simulink model "sampleModel1473"  (R2023a)
settings: Solver=VariableStepAuto  StartTime=0.0  StopTime=10.0  RelTol=1e-3
libraries: hdlsllib x6, simulink x1
settings Model: Creator=user1  LastModifiedBy=user1

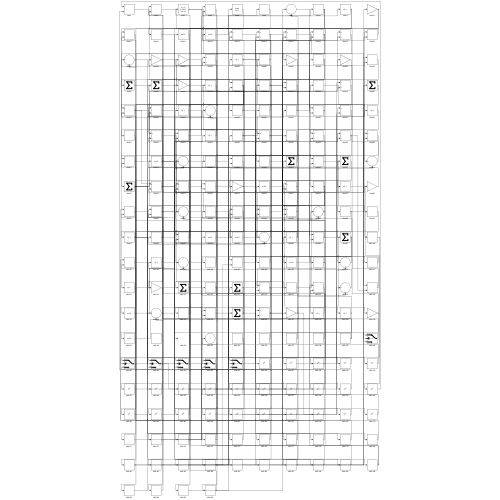
[thumbnail: Simulink's stored preview of the top-level diagram]
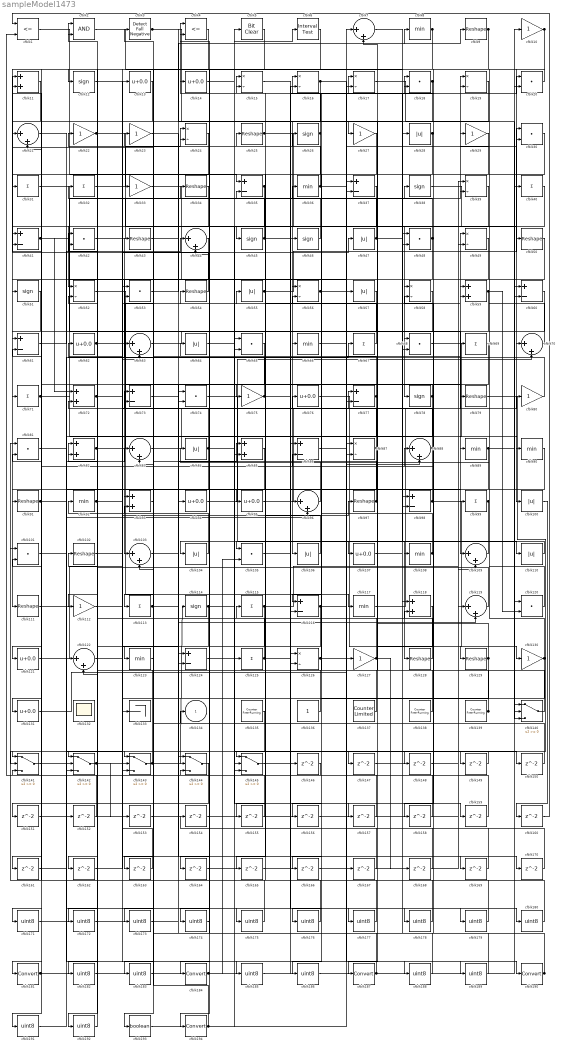
== system sampleModel1473 ==
  cfblk1 : RelationalOperator  Operator=<=  OutDataTypeStr=boolean  InputSameDT=off
  cfblk{10,22..23,27,29,33,75,80,112,127,130} (11 alike) : Gain
  cfblk{28,47,55,57,64,84,100,104,106,110} (10 alike) : Abs  SaturateOnIntegerOverflow=off
  cfblk{18,20,30,42,48,53,65,68,74,81,101,105,120} (13 alike) : DotProduct  OutDataTypeStr=Inherit: Inherit via internal rule
  cfblk{9,25,34,43,50,54,79,91,97,102,111,128..129} (13 alike) : Reshape
  cfblk{7,21,44,63,70,83,88,96,103,109,119,122} (12 alike) : Sum  Inputs=|++
  cfblk{13..14,62,76,94..95,107,121,131} (9 alike) : Bias  Bias=0.0  SaturateOnIntegerOverflow=off
  cfblk{8,36,66,89..90,92,108,117,123} (9 alike) : MinMax
  cfblk{11,59,72,82,85,93,118} (7 alike) : Sum
  cfblk{31..32,40,67,69,71,99,113,115,125} (10 alike) : Sum  Inputs=+
  cfblk{12,26,38,45..46,51,78,114} (8 alike) : Signum
  cfblk{35,37,41,60..61,73,77,86,98,116,124} (11 alike) : Sum  Inputs=+-
  cfblk{15..17,19,24,39,49,52,56,58,87,126} (12 alike) : Product  Inputs=*/  RndMeth=Zero  SaturateOnIntegerOverflow=on
  cfblk132 : Scope
      settings: Floating=on
  cfblk133 : Terminator
  cfblk135 : hdlsllib/Sources/Counter Free-Running  NumBits=16  tsamp=-1
  cfblk136 : Constant  SampleTime=-1
  cfblk137 : hdlsllib/Sources/Counter Limited  uplimit=7  tsamp=-1
  cfblk138 : hdlsllib/Sources/Counter Free-Running  NumBits=16  tsamp=-1
  cfblk139 : hdlsllib/Sources/Counter Free-Running  NumBits=16  tsamp=-1
  cfblk{140..145} (6 alike) : Switch  SaturateOnIntegerOverflow=off  InputSameDT=off
  cfblk{146..170} (25 alike) : Delay  SampleTime=1
  cfblk{171..180,182..183,185..186,188..189,191..192} (18 alike) : DataTypeConversion  OutDataTypeStr=uint8  SaturateOnIntegerOverflow=off  RndMeth=Floor
  cfblk{181,184,187,190,194} (5 alike) : DataTypeConversion  SaturateOnIntegerOverflow=off  RndMeth=Floor
  cfblk193 : DataTypeConversion  OutDataTypeStr=boolean  SaturateOnIntegerOverflow=off  RndMeth=Floor
  cfblk2 : Logic  AllPortsSameDT=off  OutDataTypeStr=boolean
  cfblk3 : hdlsllib/Logic and Bit Operations/Detect Fall Negative  vinit=0  OutDataTypeStr=boolean
  cfblk4 : RelationalOperator  Operator=<=  OutDataTypeStr=boolean  InputSameDT=off
  cfblk5 : simulink/Logic and Bit Operations/Bit Clear  iBit=0
      settings: LibrarySourceBlock=|
      | hdlsllib/Logic and Bit
      | Operations/Bit Clear
  cfblk6 : hdlsllib/Logic and Bit Operations/Interval Test  IntervalClosedRight=on  uplimit=0.5  IntervalClosedLeft=on  lowlimit=-0.5  OutDataTypeStr=boolean
  cfblk134 : Outport  VectorParamsAs1DForOutWhenUnconnected=off
  wires:
  cfblk76/1 -> cfblk129/1
  cfblk26/1 -> cfblk111/1, cfblk4/2
  cfblk110/1 -> cfblk104/1
  cfblk42/1 -> cfblk19/1
  cfblk32/1 -> cfblk24/1
  cfblk1/1 -> cfblk35/1
  cfblk8/1 -> cfblk71/1, cfblk174/1, cfblk193/1
  cfblk28/1 -> cfblk105/1, cfblk164/1
  cfblk80/1 -> cfblk43/1
  cfblk79/1 -> cfblk142/1
  cfblk72/1 -> cfblk13/1, cfblk177/1
  cfblk71/1 -> cfblk38/1, cfblk55/1, cfblk98/1, cfblk98/2
  cfblk19/1 -> cfblk106/1
  cfblk52/1 -> cfblk117/1
  cfblk139/1 -> cfblk77/1, cfblk16/1
  cfblk39/1 -> cfblk78/1
  cfblk54/1 -> cfblk11/1
  cfblk63/1 -> cfblk68/1
  cfblk44/1 -> cfblk103/1
  cfblk70/1 -> cfblk15/1
  cfblk96/1 -> cfblk22/1
  cfblk35/1 -> cfblk141/1, cfblk145/3, cfblk121/1
  cfblk29/1 -> cfblk45/1
  cfblk131/1 -> cfblk57/1
  cfblk2/1 -> cfblk48/1
  cfblk3/1 -> cfblk48/2, cfblk27/1
  cfblk14/1 -> cfblk8/1
  cfblk83/1 -> cfblk49/1
  cfblk106/1 -> cfblk15/2
  cfblk11/1 -> cfblk31/1
  cfblk85/1 -> cfblk91/1
  cfblk136/1 -> cfblk102/1
  cfblk98/1 -> cfblk130/1, cfblk11/2
  cfblk88/1 -> cfblk17/1, cfblk86/2
  cfblk77/1 -> cfblk21/1, cfblk116/2
  cfblk75/1 -> cfblk62/1, cfblk59/2, cfblk95/1
  cfblk145/1 -> cfblk46/1
  cfblk10/1 -> cfblk100/1, cfblk143/2
  cfblk97/1 -> cfblk93/1, cfblk36/1
  cfblk59/1 -> cfblk131/1, cfblk120/2
  cfblk65/1 -> cfblk181/1
  cfblk50/1 -> cfblk107/1
  cfblk87/1 -> cfblk24/2, cfblk192/1
  cfblk5/1 -> cfblk194/1
  cfblk118/1 -> cfblk187/1
  cfblk56/1 -> cfblk88/2, cfblk149/1
  cfblk58/1 -> cfblk113/1
  cfblk95/1 -> cfblk80/1
  cfblk82/1 -> cfblk54/1, cfblk76/1
  cfblk62/1 -> cfblk74/2, cfblk124/2, cfblk140/3
  cfblk78/1 -> cfblk142/2, cfblk75/1, cfblk87/2, cfblk155/1
  cfblk24/1 -> cfblk142/3
  cfblk22/1 -> cfblk127/1, cfblk112/1
  cfblk57/1 -> cfblk66/1
  cfblk143/1 -> cfblk114/1, cfblk42/2
  cfblk104/1 -> cfblk92/1
  cfblk60/1 -> cfblk184/1
  cfblk67/1 -> cfblk25/1
  cfblk41/1 -> cfblk109/1, cfblk72/1
  cfblk142/1 -> cfblk153/1, cfblk189/1
  cfblk129/1 -> cfblk7/2, cfblk156/1
  cfblk25/1 -> cfblk70/1, cfblk18/1
  cfblk114/1 -> cfblk6/1, cfblk162/1
  cfblk141/1 -> cfblk83/1
  cfblk47/1 -> cfblk19/2, cfblk34/1
  cfblk122/1 -> cfblk190/1
  cfblk33/1 -> cfblk87/1
  cfblk51/1 -> cfblk61/1
  cfblk117/1 -> cfblk10/1
  cfblk135/1 -> cfblk145/1
  cfblk130/1 -> cfblk29/1, cfblk140/2
  cfblk123/1 -> cfblk73/1
  cfblk68/1 -> cfblk90/1
  cfblk12/1 -> cfblk133/1
  cfblk102/1 -> cfblk59/1
  cfblk74/1 -> cfblk128/1
  cfblk128/1 -> cfblk63/1
  cfblk107/1 -> cfblk28/1
  cfblk17/1 -> cfblk120/1
  cfblk55/1 -> cfblk30/1, cfblk180/1
  cfblk94/1 -> cfblk70/2
  cfblk53/1 -> cfblk9/1
  cfblk34/1 -> cfblk52/1
  cfblk125/1 -> cfblk14/1, cfblk159/1
  cfblk13/1 -> cfblk51/1
  cfblk105/1 -> cfblk20/1
  cfblk73/1 -> cfblk79/1
  cfblk89/1 -> cfblk40/1, cfblk126/2
  cfblk49/1 -> cfblk58/1
  cfblk126/1 -> cfblk30/2, cfblk188/1
  cfblk138/1 -> cfblk64/1
  cfblk61/1 -> cfblk44/1
  cfblk140/1 -> cfblk26/1
  cfblk113/1 -> cfblk85/1, cfblk173/1
  cfblk92/1 -> cfblk33/1, cfblk52/2
  cfblk40/1 -> cfblk143/1
  cfblk109/1 -> cfblk108/1
  cfblk93/1 -> cfblk73/2
  cfblk119/1 -> cfblk2/1
  cfblk9/1 -> cfblk158/1, cfblk183/1
  cfblk86/1 -> cfblk69/1
  cfblk23/1 -> cfblk56/1
  cfblk116/1 -> cfblk145/2, cfblk39/2
  cfblk91/1 -> cfblk67/1, cfblk41/2, cfblk143/3, cfblk96/2
  cfblk48/1 -> cfblk23/1, cfblk191/1
  cfblk121/1 -> cfblk97/1
  cfblk18/1 -> cfblk37/2, cfblk147/1
  cfblk16/1 -> cfblk77/2, cfblk123/1, cfblk21/2
  cfblk31/1 -> cfblk126/1
  cfblk90/1 -> cfblk96/1
  cfblk7/1 -> cfblk110/1
  cfblk111/1 -> cfblk47/1
  cfblk127/1 -> cfblk82/1, cfblk168/1
  cfblk103/1 -> cfblk119/2
  cfblk20/1 -> cfblk12/1
  cfblk66/1 -> cfblk89/1
  cfblk84/1 -> cfblk42/1, cfblk150/1, cfblk151/1
  cfblk37/1 -> cfblk41/1
  cfblk38/1 -> cfblk140/1
  cfblk120/1 -> cfblk84/1
  cfblk64/1 -> cfblk56/2
  cfblk137/1 -> cfblk82/2
  cfblk108/1 -> cfblk72/2, cfblk148/1
  cfblk45/1 -> cfblk99/1, cfblk4/1
  cfblk99/1 -> cfblk165/1, cfblk166/1
  cfblk36/1 -> cfblk3/1, cfblk18/2, cfblk116/1, cfblk179/1
  cfblk115/1 -> cfblk50/1, cfblk163/1
  cfblk46/1 -> cfblk32/1
  cfblk15/1 -> cfblk146/1
  cfblk146/1 -> cfblk1/2
  cfblk147/1 -> cfblk49/2
  cfblk148/1 -> cfblk58/2
  cfblk149/1 -> cfblk141/2
  cfblk150/1 -> cfblk103/2
  cfblk151/1 -> cfblk85/2
  cfblk21/1 -> cfblk152/1
  cfblk152/1 -> cfblk141/3
  cfblk153/1 -> cfblk119/1
  cfblk154/1 -> cfblk37/1
  cfblk155/1 -> cfblk83/2
  cfblk156/1 -> cfblk68/2
  cfblk124/1 -> cfblk157/1
  cfblk157/1 -> cfblk74/1
  cfblk158/1 -> cfblk2/2
  cfblk159/1 -> cfblk61/2
  cfblk100/1 -> cfblk160/1
  cfblk160/1 -> cfblk1/1
  cfblk6/1 -> cfblk161/1
  cfblk162/1 -> cfblk63/2
  cfblk163/1 -> cfblk53/1
  cfblk164/1 -> cfblk7/1
  cfblk165/1 -> cfblk39/1
  cfblk166/1 -> cfblk109/2
  cfblk167/1 -> cfblk86/1
  cfblk168/1 -> cfblk44/2
  cfblk112/1 -> cfblk169/1
  cfblk169/1 -> cfblk88/1
  cfblk43/1 -> cfblk170/1
  cfblk170/1 -> cfblk35/2
  cfblk144/1 -> cfblk171/1
  cfblk171/1 -> cfblk94/1
  cfblk4/1 -> cfblk172/1
  cfblk172/1 -> cfblk144/1
  cfblk173/1 -> cfblk144/2
  cfblk174/1 -> cfblk144/3
  cfblk101/1 -> cfblk175/1
  cfblk175/1 -> cfblk134/1
  cfblk30/1 -> cfblk176/1
  cfblk176/1 -> cfblk101/1
  cfblk177/1 -> cfblk101/2
  cfblk81/1 -> cfblk178/1
  cfblk178/1 -> cfblk115/1
  cfblk179/1 -> cfblk81/1
  cfblk180/1 -> cfblk81/2
  cfblk181/1 -> cfblk167/1, cfblk125/1
  cfblk27/1 -> cfblk182/1
  cfblk182/1 -> cfblk65/1
  cfblk183/1 -> cfblk65/2
  cfblk184/1 -> cfblk16/2, cfblk105/2
  cfblk161/1 -> cfblk185/1
  cfblk185/1 -> cfblk60/1
  cfblk69/1 -> cfblk186/1
  cfblk186/1 -> cfblk60/2
  cfblk187/1 -> cfblk154/1, cfblk20/2
  cfblk188/1 -> cfblk118/1
  cfblk189/1 -> cfblk118/2
  cfblk190/1 -> cfblk53/2, cfblk124/1
  cfblk191/1 -> cfblk122/1
  cfblk192/1 -> cfblk122/2
  cfblk193/1 -> cfblk5/1
  cfblk194/1 -> cfblk17/2, cfblk93/2
